simulink model "model"  (R2019b)
settings: Solver=VariableStepAuto  StartTime=0.0  StopTime=50.0  RelTol=1e-3
values from neighbouring files (symbols this model uses):
  Kkr = 8    [zad1.m]    (also in zad1_m.m)
  Pkr = 3.5    [zad1.m]    (also in zad1_m.m)
settings Model: Creator=marci  LastModifiedBy=marci

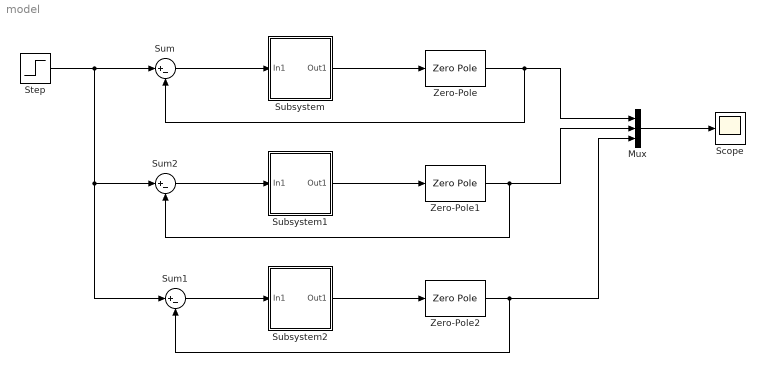
== system model ==
  Mux : Mux  Inputs=3
  Scope : Scope
  Step : Step  SampleTime=0
  Subsystem : Subsystem  mask{P=0.5* Kkr, I=10000, D=0}
  Subsystem1 : Subsystem  mask{P=0.45* Kkr, I=Pkr/1.2, D=0}
  Subsystem2 : Subsystem  mask{P=0.6* Kkr, I=Pkr/2, D=Pkr/8}
  Sum : Sum  Inputs=|+-
  Sum1 : Sum  Inputs=|+-
  Sum2 : Sum  Inputs=|+-
  Zero-Pole : ZeroPole  Zeros=[]  Poles=[-1 -1 -1]
  Zero-Pole1 : ZeroPole  Zeros=[]  Poles=[-1 -1 -1]
  Zero-Pole2 : ZeroPole  Zeros=[]  Poles=[-1 -1 -1]
  wires:
  Step/1 -> Sum1/1, Sum2/1, Sum/1
  Sum/1 -> Subsystem/1(In1)
  Subsystem/1(Out1) -> Zero-Pole/1
  Zero-Pole/1 -> Sum/2, Mux/1
  Sum2/1 -> Subsystem1/1(In1)
  Subsystem1/1(Out1) -> Zero-Pole1/1
  Zero-Pole1/1 -> Mux/2, Sum2/2
  Sum1/1 -> Subsystem2/1(In1)
  Subsystem2/1(Out1) -> Zero-Pole2/1
  Zero-Pole2/1 -> Mux/3, Sum1/2
  Mux/1 -> Scope/1

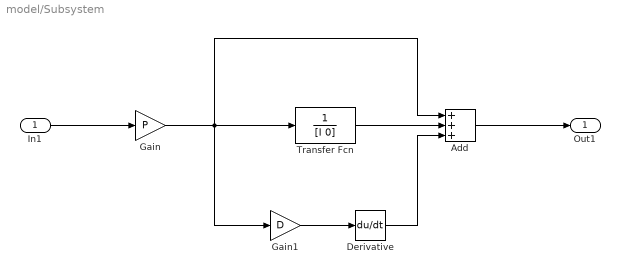
== system model/Subsystem ==
  In1 : Inport
  Add : Sum  Inputs=+++
  Derivative : Derivative
  Gain : Gain  Gain=P
  Gain1 : Gain  Gain=D
  Transfer Fcn : TransferFcn  Denominator=[I 0]
  Out1 : Outport
  wires:
  Add/1 -> Out1/1
  Gain1/1 -> Derivative/1
  In1/1 -> Gain/1
  Derivative/1 -> Add/3
  Transfer Fcn/1 -> Add/2
  Gain/1 -> Gain1/1, Transfer Fcn/1, Add/1

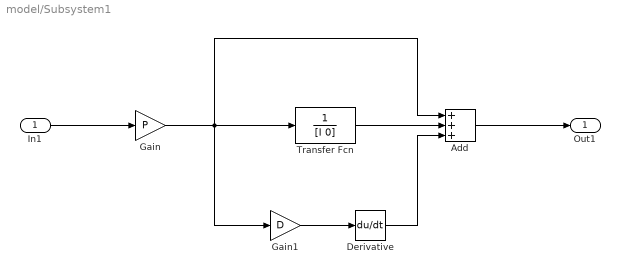
== system model/Subsystem1 ==
  In1 : Inport
  Add : Sum  Inputs=+++
  Derivative : Derivative
  Gain : Gain  Gain=P
  Gain1 : Gain  Gain=D
  Transfer Fcn : TransferFcn  Denominator=[I 0]
  Out1 : Outport
  wires:
  Add/1 -> Out1/1
  Gain1/1 -> Derivative/1
  In1/1 -> Gain/1
  Derivative/1 -> Add/3
  Transfer Fcn/1 -> Add/2
  Gain/1 -> Gain1/1, Transfer Fcn/1, Add/1

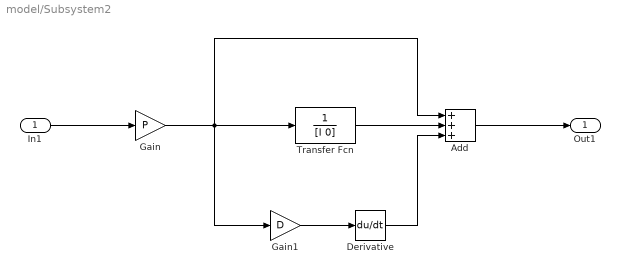
== system model/Subsystem2 ==
  In1 : Inport
  Add : Sum  Inputs=+++
  Derivative : Derivative
  Gain : Gain  Gain=P
  Gain1 : Gain  Gain=D
  Transfer Fcn : TransferFcn  Denominator=[I 0]
  Out1 : Outport
  wires:
  Add/1 -> Out1/1
  Gain1/1 -> Derivative/1
  In1/1 -> Gain/1
  Derivative/1 -> Add/3
  Transfer Fcn/1 -> Add/2
  Gain/1 -> Gain1/1, Transfer Fcn/1, Add/1
